simulink model "Part3"  (R2020a)
settings: Solver=VariableStepAuto  StartTime=0.0  StopTime=inf  RelTol=1e-3
values from neighbouring files (symbols this model uses):
  b = 50    [Script1.m]
  m = 1000    [Script1.m]
  Te = 3/5    (= 0.6)    [Script1.m]
libraries: cstblocks x1
settings Model: Creator=maxen  LastModifiedBy=maxen

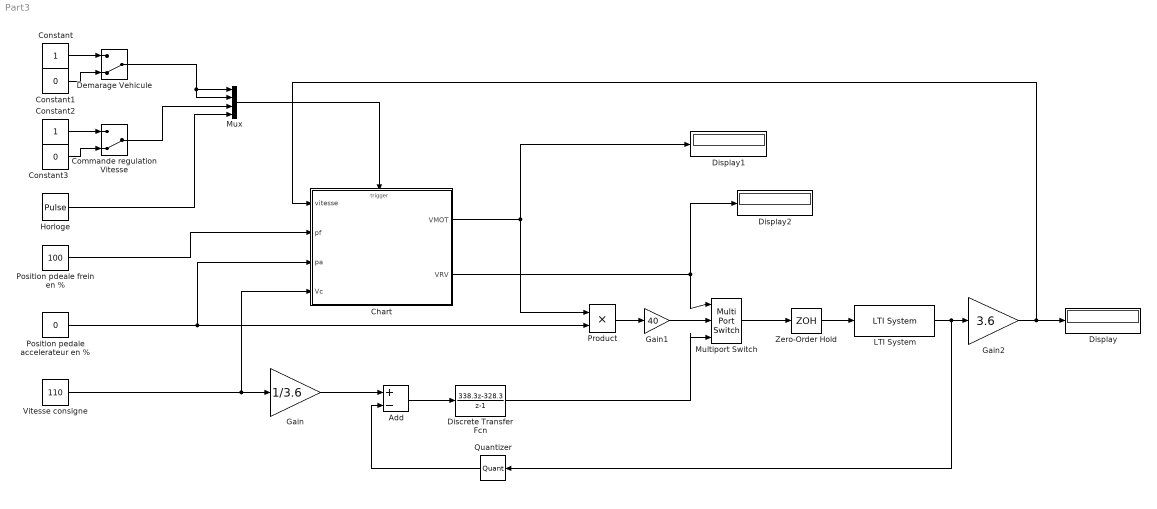
== system Part3 ==
  Add : Sum  Inputs=+-
  Chart : Stateflow chart  TreatAsAtomicUnit=on
  Commande regulation Vitesse : ManualSwitch  CurrentSetting=0
  Constant : Constant
  Constant1 : Constant  Value=0
  Constant2 : Constant
  Constant3 : Constant  Value=0
  Demarage Vehicule : ManualSwitch  CurrentSetting=0
  Discrete Transfer Fcn : DiscreteTransferFcn  Numerator=[338.3 -328.3]  Denominator=[1 -1]  SampleTime=0.6
  Display : Display
  Display1 : Display
  Display2 : Display
  Gain : Gain  Gain=1/3.6
  Gain1 : Gain  Gain=40
  Gain2 : Gain  Gain=3.6
  Horloge : DiscretePulseGenerator  PulseType=Time based  Period=0.1  PulseWidth=50
  LTI System : cstblocks/LTI System  sys=tf(1,[m b])  IC=[]
  Multiport Switch : MultiPortSwitch  Inputs=2
  Mux : Mux
  Position pdeale frein en % : Constant  Value=100
  Position pedale accelerateur en % : Constant  Value=0
  Product : Product
  Quantizer : Quantizer  QuantizationInterval=0.25
  Vitesse consigne : Constant  Value=110
  Zero-Order Hold : ZeroOrderHold  SampleTime=Te
  wires:
  Constant1/1 -> Demarage Vehicule/2
  Constant/1 -> Demarage Vehicule/1
  Constant2/1 -> Commande regulation Vitesse/1
  Constant3/1 -> Commande regulation Vitesse/2
  Commande regulation Vitesse/1 -> Mux/3
  Demarage Vehicule/1 -> Mux/2, Mux/1
  Horloge/1 -> Mux/4
  Position pdeale frein en %/1 -> Chart/2(pf)
  Position pedale accelerateur en %/1 -> Chart/3(pa), Product/2
  Vitesse consigne/1 -> Chart/4(Vc), Gain/1
  Add/1 -> Discrete Transfer Fcn/1
  Gain/1 -> Add/1
  Product/1 -> Gain1/1
  Gain1/1 -> Multiport Switch/2
  Discrete Transfer Fcn/1 -> Multiport Switch/3
  Multiport Switch/1 -> Zero-Order Hold/1
  Zero-Order Hold/1 -> LTI System/1
  LTI System/1 -> Quantizer/1, Gain2/1
  Quantizer/1 -> Add/2
  Gain2/1 -> Chart/1(vitesse), Display/1
  Mux/1 -> Chart/Trigger
  Chart/1(VMOT) -> Display1/1, Product/1
  Chart/2(VRV) -> Display2/1, Multiport Switch/1

== stateflow chart Part3/Chart ==
  state X0
  state X2
    en:VMOT=1;
    en:VRV=1;
  state X1_ATTENTE
  state X3
    en:VRV=2;
  state X4
    en:VRV=1;
  state X5
    en:VMOT=0;
  (default) -> X0
  X5 -> X0
  X0 -> X2 : contact_ON
  X2 -> (junction 13)
  (junction 13) -> (junction 25) [order 2]
  (junction 13) -> X1_ATTENTE [order 1] : mrv_bouton[(vitesse>80) & ((Vc-vitesse)<30)]
  X1_ATTENTE -> X3 : after(100,horloge)
  X3 -> X4 [order 3] : mrv_bouton
  X3 -> X4 [order 1] : [pf>0]
  X3 -> X4 [order 2] : [pa == 100]
  X4 -> (junction 25)
  (junction 25) -> X5 : contact_OFF[vitesse<1]
  data: VMOT output double; vitesse input double; pf input double; pa input double; Vc input double; VRV output double =1
  events: contact_ON input RISING_EDGE_EVENT; contact_OFF input FALLING_EDGE_EVENT; mrv_bouton input EITHER_EDGE_EVENT; horloge input RISING_EDGE_EVENT
